simulink model "model_virtualagent_bros"  (R2016b)
settings: Solver=FixedStepDiscrete  StartTime=0.0  StopTime=inf  FixedStep=sampleTime  RelTol=1e-3
PostLoadFcn:
  | % load model parameters
  | % pname = fileparts(get_param('model_virtualagent_bros','filename'));
  | % run([pname  '\parameters_base_model_bros.m']);
  | parameters_base_model_bros;
  | 
  | % set requested state
  | set_param('model_virtualagent_bros/Requested state','Value',num2str(0));
InitFcn:
  | % load model parameters
  | % pname = fileparts(get_param('model_base_bros','filename'));
  | % run([pname  '\parameters_base_model_bros.m']);
  | parameters_base_model_bros;
  | 
  | % set requested state
  | set_param('model_virtualagent_bros/Requested state','Value',num2str(0));
StartFcn:
  | % load model parameters
  | % pname = fileparts(get_param('model_base_bros','filename'));
  | % run([pname  '\parameters_base_model_bros.m']);
  | parameters_base_model_bros;
  | 
  | % set requested state
  | set_param('model_virtualagent_bros/Requested state','Value',num2str(0));
values from neighbouring files (symbols this model uses):
  Ae_vp = [1 2;3 4]    [parameters_base_model_bros.m]
  Aim_vp = Ae_vp    [parameters_base_model_bros.m]    (also in parameters_virtualpartner_bros.m = dynamics_vp(sampleTime,m_vp,tu,td,tp,gamma*D))
  Ax = [0.0286583637244 0.0270981680387 0.0234505258969 0.0179991434705]    [data_target_signal.mat]    (also in data_target_signal3.mat = [0.0333782282668 0.0245436264839 0.0161138842629 0.007570500; data_target_signal4.mat = [0.0269405878553 0.022932388404 0.0177213023263 0.0101459636; data_target_signal5.mat = [0.0280601816416 0.0238854099083 0.0184577621273 0.010567608)
  Ay = [0.0270981680387 0.0253254894496 0.0215637914741 0.0163904070646]    [data_target_signal.mat]    (also in data_target_signal3.mat = [0.0316365733513 0.022903298684 0.0150378639378 0.0071644979; data_target_signal4.mat = [0.0262391735578 0.0220449066546 0.0169202788634 0.009702651; data_target_signal5.mat = [0.0273296180511 0.0229610462966 0.0176234498254 0.010105872)
  FFMatrix = [0 -20; 20 0]*-1    [parameters_base_model_bros.m]    (also in parameters_model_virtualpartner_bros.m = -[0 -15; 15 0]; parameters_virtualpartner_bros.m = -[0 -15; 15 0])
  Lb = 0.07    [parameters_base_model_bros.m]    (also in parameters_model_virtualpartner_bros.m; parameters_virtualpartner_bros.m)
  Lf = 0.238    [parameters_base_model_bros.m]    (also in parameters_model_virtualpartner_bros.m; parameters_virtualpartner_bros.m)
  Lu = 0.153    [parameters_base_model_bros.m]    (also in parameters_model_virtualpartner_bros.m; parameters_virtualpartner_bros.m)
  nx = [3 4 6 9]    [data_target_signal.mat]    (also in data_target_signal3.mat = [6 11 17 29]; data_target_signal4.mat = [6 11 17 29]; data_target_signal5.mat = [6 11 17 29])
  ny = [4 5 7 10]    [data_target_signal.mat]    (also in data_target_signal3.mat = [7 12 18 30]; data_target_signal4.mat = [7 12 18 30]; data_target_signal5.mat = [7 12 18 30])
  P0_vp = zeros(2,2)    [parameters_base_model_bros.m]
  phx = [-7.77441521106 -8.5348832042 -4.36104325862 -3.78796037329]    [data_target_signal.mat]    (also in data_target_signal3.mat = [3.56575266464 -2.00335535647 1.65538939475 0.759048650391]; data_target_signal4.mat = [-7.8125213649 -4.12353525545 6.3256632478 -1.21163926456]; data_target_signal5.mat = [2.80153374524 -3.20046313064 -3.48286348128 -10.5236026319])
  phy = [-0.714244784373 -3.45250659197 3.9180169666 4.93073057512]    [data_target_signal.mat]    (also in data_target_signal3.mat = [9.98760310067 -6.16453798136 -6.84315611985 5.69872885715]; data_target_signal4.mat = [6.54917483844 9.11210927212 4.8993819932 2.56946947623]; data_target_signal5.mat = [-1.40862004251 -1.67034924642 8.20266618674 -4.37156725072])
  sampleTime = 0.001    [parameters_base_model_bros.m]    (also in parameters_model_virtualpartner_bros.m; parameters_virtualpartner_bros.m)
undefined symbols (not defined in the file or in its folder): B_vp, BROS1, BROS2, C_vp
libraries: simulink x26, LibraryFM x14, VariousBlocksLibrary x6, simulink_extras x1
(part 3 of 3)

== system model_virtualagent_bros/Robot1/DataFromEtherCAT/Calculate Arrange Joint and Op Space/forward kinematics1 ==
  JointPosition_rad : Inport  PortDimensions=[2 1]
  JointVelocity_rads : Inport  Port=2  PortDimensions=[2 1]
  JointAcceleration_rads2 : Inport  Port=3  PortDimensions=[2 1]
  Je : MATLAB Function  TreatAsAtomicUnit=on
  Jedot : MATLAB Function  TreatAsAtomicUnit=on
  Product : Product  Multiplication=Matrix(*)
  calculate xddot : MATLAB Function  TreatAsAtomicUnit=on
  forward kinematics : MATLAB Function  TreatAsAtomicUnit=on
  x : Outport
  xdot : Outport  Port=2
  xddot : Outport  Port=3
  J : Outport  Port=4
  Jdot : Outport  Port=5
  wires:
  JointPosition_rad/1 -> forward kinematics/1(q), Jedot/1(q), Je/1(q)
  Je/1(Je) -> calculate xddot/3(J), Product/1, J/1
  JointVelocity_rads/1 -> calculate xddot/2(qdot), Product/2, Jedot/2(qdot)
  Jedot/1(Jedot) -> calculate xddot/4(Jdot), Jdot/1
  Product/1 -> xdot/1
  forward kinematics/1(x) -> x/1
  calculate xddot/1(xddot) -> xddot/1
  JointAcceleration_rads2/1 -> calculate xddot/1(qddot)

== system model_virtualagent_bros/Robot2/Controller_PD/at home/HoldFirstSampleOnEnable ==
  note: These blocks hold the first sample of the input
      | when the block is enabled (through the action port)
  x : Inport
  Enable : EnablePort  StatesWhenEnabling=reset
  Counter Free-Running : simulink/Sources/Counter Free-Running  NumBits=32  tsamp=-1
  Memory1 : Memory
  Signal Conversion : SignalConversion  OverrideOpt=off
  Switch : Switch  Threshold=1
  x0 : Outport
  wires:
  x/1 -> Switch/3
  Counter Free-Running/1 -> Switch/2
  Memory1/1 -> Switch/1
  Switch/1 -> Signal Conversion/1, Memory1/1
  Signal Conversion/1 -> x0/1

== system model_virtualagent_bros/Robot2/DataFromEtherCAT/Calculate Arrange Joint and Op Space/forward kinematics ==
  JointPosition_rad : Inport  PortDimensions=[2 1]
  JointVelocity_rads : Inport  Port=2  PortDimensions=[2 1]
  JointAcceleration_rads2 : Inport  Port=3  PortDimensions=[2 1]
  Je : MATLAB Function  TreatAsAtomicUnit=on
  Jedot : MATLAB Function  TreatAsAtomicUnit=on
  Product : Product  Multiplication=Matrix(*)
  calculate xddot : MATLAB Function  TreatAsAtomicUnit=on
  forward kinematics : MATLAB Function  TreatAsAtomicUnit=on
  x : Outport
  xdot : Outport  Port=2
  xddot : Outport  Port=3
  J : Outport  Port=4
  Jdot : Outport  Port=5
  wires:
  JointPosition_rad/1 -> forward kinematics/1(q), Jedot/1(q), Je/1(q)
  Je/1(Je) -> calculate xddot/3(J), Product/1, J/1
  JointVelocity_rads/1 -> calculate xddot/2(qdot), Product/2, Jedot/2(qdot)
  Jedot/1(Jedot) -> calculate xddot/4(Jdot), Jdot/1
  Product/1 -> xdot/1
  forward kinematics/1(x) -> x/1
  calculate xddot/1(xddot) -> xddot/1
  JointAcceleration_rads2/1 -> calculate xddot/1(qddot)

== system model_virtualagent_bros/Robot2/DataFromEtherCAT/Calculate Arrange Joint and Op Space/forward kinematics1 ==
  JointPosition_rad : Inport  PortDimensions=[2 1]
  JointVelocity_rads : Inport  Port=2  PortDimensions=[2 1]
  JointAcceleration_rads2 : Inport  Port=3  PortDimensions=[2 1]
  Je : MATLAB Function  TreatAsAtomicUnit=on
  Jedot : MATLAB Function  TreatAsAtomicUnit=on
  Product : Product  Multiplication=Matrix(*)
  calculate xddot : MATLAB Function  TreatAsAtomicUnit=on
  forward kinematics : MATLAB Function  TreatAsAtomicUnit=on
  x : Outport
  xdot : Outport  Port=2
  xddot : Outport  Port=3
  J : Outport  Port=4
  Jdot : Outport  Port=5
  wires:
  JointPosition_rad/1 -> forward kinematics/1(q), Jedot/1(q), Je/1(q)
  Je/1(Je) -> calculate xddot/3(J), Product/1, J/1
  JointVelocity_rads/1 -> calculate xddot/2(qdot), Product/2, Jedot/2(qdot)
  Jedot/1(Jedot) -> calculate xddot/4(Jdot), Jdot/1
  Product/1 -> xdot/1
  forward kinematics/1(x) -> x/1
  calculate xddot/1(xddot) -> xddot/1
  JointAcceleration_rads2/1 -> calculate xddot/1(qddot)

== matlab function model_virtualagent_bros/Robot2/Controller_PD/PD + nonlin (op space)/Jt ==
  data: x input; J input; y output
function y = Jt(x,J)

y = J.'*x;

== matlab function model_virtualagent_bros/Experiment & Haptics/CalculateTrialPerformanceMSE/Calc_RMSE_BROS1 ==
  data: error input; RMSE output
function RMSE = RMSE(error)
% calculate the mean-squared error

persistent N; % number of samples, counter
persistent SSE; % sum of squared of error
if isempty(N), N = 0; end
if isempty(SSE), SSE = 0; end

N = N+1; % new datapoint, increase sample counter

SSE = SSE + norm(error)^2;
RMSE = sqrt(SSE / N);

== matlab function model_virtualagent_bros/Robot1/DataFromEtherCAT/Calculate Arrange Joint and Op Space/Condition number ==
  data: J input; C output
function C = conditioning(J)
%#codegen

C = norm(J)*norm(pinv(J));

== matlab function model_virtualagent_bros/Robot1/DataFromEtherCAT/Calculate Arrange Joint and Op Space/forward kinematics1/Je ==
  data: q input; Je output size=[2 2]; Lf parameter; Lu parameter; Lb parameter
function Je = Je( q, Lf, Lu, Lb)
%#codegen

% Calculate the Jacobian for this particular device configuration.
% Note that the function func_eq_Je needs to be in the libraries/kinematis_functions folder

% jacobians
Je = func_eq_Je(q(1),q(2),Lf,Lu,Lb);

== matlab function model_virtualagent_bros/Robot1/DataFromEtherCAT/Calculate Arrange Joint and Op Space/forward kinematics1/Jedot ==
  data: q input; qdot input; Jedot output size=[2 2]; Lf parameter; Lu parameter; Lb parameter
function Jedot = Jedot( q, qdot, Lf, Lu, Lb)
%#codegen

% Calculate the time derivative of the Jacobian for this particular device configuration.
% Note that the function func_eq_Je needs to be in the libraries/kinematis_functions folder


% jacobians
Jedot = func_eq_Jedot(q(1),q(2),qdot(1),qdot(2),Lf,Lu,Lb);

== matlab function model_virtualagent_bros/Robot1/DataFromEtherCAT/Calculate Arrange Joint and Op Space/forward kinematics1/calculate xddot ==
  data: qddot input; qdot input size=[2 1]; J input; xddot output size=[2 1]; Jdot input
function xddot = calc_xddot(qddot, qdot, J, Jdot)
%#codegen

xddot = J*qddot + Jdot*qdot;

== matlab function model_virtualagent_bros/Robot2/Controller_PD/PD + nonlin (op space)/nonlinear compensation ==
  data: J input; Jdot input; qdot input; tau output; RobotStruct parameter
function tau = n(J,Jdot,qdot,RobotStruct)
% mass matrix
phat = RobotStruct.DynModParams;

% select parameters
me = phat(3);
Fs1 = phat(4);
Fv1 = phat(5);
Fs2 = phat(6);
Fv2 = phat(7);

% % jacobians
% J = func_eq_Je(q(1),q(2),Lf,Lu,Lb);
% Jdot = func_eq_Jedot(q(1),q(2),qdot(1),qdot(2),Lf,Lu,Lb);

% calculate joint space mass matrix;
p = [me;Fs1;Fv1;Fs2;Fv2];

% psi 
Psi = [(J'*Jdot)*qdot [ssign(qdot(1)) qdot(1); 0 0] [0 0; ssign(qdot(2)) qdot(2)]];

% torque
tau = Psi*p;

function x = ssign(u,b)
%% x = ssign(u,b)
% soft sign
if nargin < 2
    b = 4;
end

x = 2./(1+exp(-b*u))-1;

== matlab function model_virtualagent_bros/Experiment & Haptics/Target position ==
  data: time input; T input; time_rand input; p output; nx parameter; ny parameter; Ax parameter; Ay parameter; phx parameter; phy parameter
function p  = msin_target (time, T, time_rand, nx, ny, Ax, Ay, phx, phy) 

% prepare frequencies
dw = 2*pi/T; %w0 depends on trial duration
wx = dw*nx;
wy = dw*ny;

% calculate x and y
px = 0;
py = 0;

% randomization
% for every multiple of 20, mirror x, y, or xy
% nRand = 0: no mirror
% nRand = 1: x mirror
% nRand = 2: y mirror
% nRand = 3: xy mirror
nRand = floor(time_rand/20);
if nRand > 3, nRand = 3; end

% add random starting time (semi-randomization)
time = time + mod(time_rand,20.0);

% calculate sum-of-sines
for i = 1:length(wx)
    px = px + Ax(i)*sin(wx(i)*time+phx(i));
    py = py + Ay(i)*sin(wy(i)*time+phy(i));
end

p = [px; py];

% mirror position, based on nRand
switch nRand
    case 0
        % do nothing
    case 1
        p = [-1;1].*p;
    case 2
        p = [1;-1].*p;
    case 3
        p = [-1;-1].*p;
    otherwise
        % do nothing
end
end

== matlab function model_virtualagent_bros/Robot1/DataFromEtherCAT/Calculate Arrange Joint and Op Space/forward kinematics/forward kinematics ==
  data: q input; x output size=[2 1]; Lf parameter; Lu parameter; Lb parameter
function x = FK(q, Lf, Lu, Lb)
%#codegen

% Calculate the endpoint position (forward kinematics)
% Note that the function func_eq_FK needs to be in the libraries/kinematis_functions folder


x = func_eq_FK(q(1),q(2),Lf,Lu,Lb);

== matlab function model_virtualagent_bros/Robot1/DataFromEtherCAT/Calculate Arrange Joint and Op Space/forward kinematics1/forward kinematics ==
  data: q input; x output size=[2 1]; Lf parameter; Lu parameter; Lb parameter
function x = FK(q, Lf, Lu, Lb)
%#codegen

% Calculate the endpoint position (forward kinematics)
% Note that the function func_eq_FK needs to be in the libraries/kinematis_functions folder


x = func_eq_FK(q(1),q(2),Lf,Lu,Lb);

== matlab function model_virtualagent_bros/Robot1/DataToEtherCAT/FTSensorError/MATLAB Function ==
  data: ForcesTorques input; e output; MaxForcesTorques input
function e = fcn(ForcesTorques, MaxForcesTorques)

% throw error when any of the forces/torques go over a max allowable value
if any(abs(ForcesTorques) > MaxForcesTorques) 
    e = 1;
else
    e = 0;
end

== matlab function model_virtualagent_bros/Robot1/Controller_PD/PD + nonlin (op space)/invJ1 ==
  data: x input; J input; y output
function y = invJ(x,J)

y = J.'*x;

== matlab function model_virtualagent_bros/Robot2/DataFromEtherCAT/Calculate Arrange Joint and Op Space/Condition number ==
  data: J input; C output
function C = conditioning(J)
%#codegen

C = norm(J)*norm(pinv(J));

== matlab function model_virtualagent_bros/Robot2/DataFromEtherCAT/Calculate Arrange Joint and Op Space/IK all joints ==
  data: x input; q_all output; Lf parameter; Lu parameter; Lb parameter
function q_all = IK_all(x,Lf,Lu,Lb)
%#codegen

q_all = func_eqs_IK_all(x(1),x(2),Lf,Lu,Lb);

if any(isnan(q_all)) || any(isinf(q_all))
    q_all = zeros(5,1);
end

== matlab function model_virtualagent_bros/Robot2/DataFromEtherCAT/Calculate Arrange Joint and Op Space/forward kinematics/Je ==
  data: q input; Je output size=[2 2]; Lf parameter; Lu parameter; Lb parameter
function Je = Je( q, Lf, Lu, Lb)
%#codegen

% Calculate the Jacobian for this particular device configuration.
% Note that the function func_eq_Je needs to be in the libraries/kinematis_functions folder

% jacobians
Je = func_eq_Je(q(1),q(2),Lf,Lu,Lb);

== matlab function model_virtualagent_bros/Robot2/DataFromEtherCAT/Calculate Arrange Joint and Op Space/forward kinematics/Jedot ==
  data: q input; qdot input; Jedot output size=[2 2]; Lf parameter; Lu parameter; Lb parameter
function Jedot = Jedot( q, qdot, Lf, Lu, Lb)
%#codegen

% Calculate the time derivative of the Jacobian for this particular device configuration.
% Note that the function func_eq_Je needs to be in the libraries/kinematis_functions folder


% jacobians
Jedot = func_eq_Jedot(q(1),q(2),qdot(1),qdot(2),Lf,Lu,Lb);

== matlab function model_virtualagent_bros/Robot1/DataFromEtherCAT/Calculate Arrange Joint and Op Space/forward kinematics/Je ==
  data: q input; Je output size=[2 2]; Lf parameter; Lu parameter; Lb parameter
function Je = Je( q, Lf, Lu, Lb)
%#codegen

% Calculate the Jacobian for this particular device configuration.
% Note that the function func_eq_Je needs to be in the libraries/kinematis_functions folder

% jacobians
Je = func_eq_Je(q(1),q(2),Lf,Lu,Lb);

== matlab function model_virtualagent_bros/Robot1/DataFromEtherCAT/Calculate Arrange Joint and Op Space/forward kinematics/Jedot ==
  data: q input; qdot input; Jedot output size=[2 2]; Lf parameter; Lu parameter; Lb parameter
function Jedot = Jedot( q, qdot, Lf, Lu, Lb)
%#codegen

% Calculate the time derivative of the Jacobian for this particular device configuration.
% Note that the function func_eq_Je needs to be in the libraries/kinematis_functions folder


% jacobians
Jedot = func_eq_Jedot(q(1),q(2),qdot(1),qdot(2),Lf,Lu,Lb);

== matlab function model_virtualagent_bros/Robot1/DataFromEtherCAT/FTSensor_K6D27/CorrectOffset ==
  data: u_in input; u_out output; reset input; corrected output
function [u_out,corrected] = CorrectOffset(u_in,reset)
%#codegen

persistent data_ offset_ counter_ corrected_;
N = 1000;

% initialize
if isempty(data_)
    data_ = zeros(size(u_in,1), N);
    offset_ = zeros(size(u_in));
    counter_ = 1;
    corrected_ = 0;
end

if (counter_ <= N)
    data_(:,counter_) = u_in;
end

counter_ = counter_ + 1;
if reset
    counter_ = 1;
end

% calculate mean
if counter_ == N
    corrected_ = 1;
    offset_ = mean(data_,2);
end

corrected = corrected_;
u_out = u_in - offset_;

== matlab function model_virtualagent_bros/Robot2/DataFromEtherCAT/Calculate Arrange Joint and Op Space/forward kinematics/calculate xddot ==
  data: qddot input; qdot input size=[2 1]; J input; xddot output size=[2 1]; Jdot input
function xddot = calc_xddot(qddot, qdot, J, Jdot)
%#codegen

xddot = J*qddot + Jdot*qdot;

== matlab function model_virtualagent_bros/Robot1/DataFromEtherCAT/Calculate Arrange Joint and Op Space/IK all joints ==
  data: x input; q_all output; Lf parameter; Lu parameter; Lb parameter
function q_all = IK_all(x,Lf,Lu,Lb)
%#codegen

q_all = func_eqs_IK_all(x(1),x(2),Lf,Lu,Lb);

if any(isnan(q_all)) || any(isinf(q_all))
    q_all = zeros(5,1);
end

== matlab function model_virtualagent_bros/Robot1/DataFromEtherCAT/Calculate Arrange Joint and Op Space/forward kinematics/calculate xddot ==
  data: qddot input; qdot input size=[2 1]; J input; xddot output size=[2 1]; Jdot input
function xddot = calc_xddot(qddot, qdot, J, Jdot)
%#codegen

xddot = J*qddot + Jdot*qdot;

== matlab function model_virtualagent_bros/Robot2/DataFromEtherCAT/Calculate Arrange Joint and Op Space/forward kinematics/forward kinematics ==
  data: q input; x output size=[2 1]; Lf parameter; Lu parameter; Lb parameter
function x = FK(q, Lf, Lu, Lb)
%#codegen

% Calculate the endpoint position (forward kinematics)
% Note that the function func_eq_FK needs to be in the libraries/kinematis_functions folder


x = func_eq_FK(q(1),q(2),Lf,Lu,Lb);

== matlab function model_virtualagent_bros/Robot1/Controller_PD/PD + nonlin (op space)/nonlinear compensation ==
  data: J input; Jdot input; qdot input; tau output; RobotStruct parameter
function tau = n(J,Jdot,qdot,RobotStruct)
% mass matrix
phat = RobotStruct.DynModParams;

% select parameters
me = phat(3);
Fs1 = phat(4);
Fv1 = phat(5);
Fs2 = phat(6);
Fv2 = phat(7);

% % jacobians
% J = func_eq_Je(q(1),q(2),Lf,Lu,Lb);
% Jdot = func_eq_Jedot(q(1),q(2),qdot(1),qdot(2),Lf,Lu,Lb);

% calculate joint space mass matrix;
p = [me;Fs1;Fv1;Fs2;Fv2];

% psi 
Psi = [(J'*Jdot)*qdot [ssign(qdot(1)) qdot(1); 0 0] [0 0; ssign(qdot(2)) qdot(2)]];

% torque
tau = Psi*p;

function x = ssign(u,b)
%% x = ssign(u,b)
% soft sign
if nargin < 2
    b = 8;
end

x = 2./(1+exp(-b*u))-1;

== matlab function model_virtualagent_bros/Robot2/DataFromEtherCAT/Calculate Arrange Joint and Op Space/forward kinematics1/Je ==
  data: q input; Je output size=[2 2]; Lf parameter; Lu parameter; Lb parameter
function Je = Je( q, Lf, Lu, Lb)
%#codegen

% Calculate the Jacobian for this particular device configuration.
% Note that the function func_eq_Je needs to be in the libraries/kinematis_functions folder

% jacobians
Je = func_eq_Je(q(1),q(2),Lf,Lu,Lb);

== matlab function model_virtualagent_bros/Robot2/DataFromEtherCAT/Calculate Arrange Joint and Op Space/forward kinematics1/Jedot ==
  data: q input; qdot input; Jedot output size=[2 2]; Lf parameter; Lu parameter; Lb parameter
function Jedot = Jedot( q, qdot, Lf, Lu, Lb)
%#codegen

% Calculate the time derivative of the Jacobian for this particular device configuration.
% Note that the function func_eq_Je needs to be in the libraries/kinematis_functions folder


% jacobians
Jedot = func_eq_Jedot(q(1),q(2),qdot(1),qdot(2),Lf,Lu,Lb);

== matlab function model_virtualagent_bros/Robot2/DataFromEtherCAT/Calculate Arrange Joint and Op Space/forward kinematics1/calculate xddot ==
  data: qddot input; qdot input size=[2 1]; J input; xddot output size=[2 1]; Jdot input
function xddot = calc_xddot(qddot, qdot, J, Jdot)
%#codegen

xddot = J*qddot + Jdot*qdot;

== matlab function model_virtualagent_bros/Robot2/DataFromEtherCAT/Calculate Arrange Joint and Op Space/forward kinematics1/forward kinematics ==
  data: q input; x output size=[2 1]; Lf parameter; Lu parameter; Lb parameter
function x = FK(q, Lf, Lu, Lb)
%#codegen

% Calculate the endpoint position (forward kinematics)
% Note that the function func_eq_FK needs to be in the libraries/kinematis_functions folder


x = func_eq_FK(q(1),q(2),Lf,Lu,Lb);

== matlab function model_virtualagent_bros/Robot2/DataFromEtherCAT/FTSensor_K6D27/CorrectOffset ==
  data: u_in input; u_out output; reset input; corrected output
function [u_out,corrected] = CorrectOffset(u_in,reset)
%#codegen

persistent data_ offset_ counter_ corrected_;
N = 1000;

% initialize
if isempty(data_)
    data_ = zeros(size(u_in,1), N);
    offset_ = zeros(size(u_in));
    counter_ = 1;
    corrected_ = 0;
end

if (counter_ <= N)
    data_(:,counter_) = u_in;
end

counter_ = counter_ + 1;
if reset
    counter_ = 1;
end

% calculate mean
if counter_ == N
    corrected_ = 1;
    offset_ = mean(data_,2);
end

corrected = corrected_;
u_out = u_in - offset_;

== matlab function model_virtualagent_bros/Robot2/DataFromEtherCAT/FTSensor_K6D27/SensorToOperationalSpace ==
  data: q_all input; Fs input; FTOpSpace output; transmatside input
function FTOpSpace = ForceSensorToOperationalSpace(q_all,Fs,transmatside)
%#codegen
q1 = q_all(1);
q2 = q_all(2);
q4 = q_all(4);
q5 = q_all(5);

% based on which arm the force sensor is connected
switch transmatside
    case 1
        alpha = pi-q2;   
        beta = q1+alpha-pi/2;
        R0 = rotmat(beta);
        R = blkdiag(R0,R0); % transform forces and moments
    case 2
        alpha = -(pi - q4);
        beta = q5+alpha-pi/2;
        R0 = rotmat(beta);
        R = blkdiag(R0,R0); % transform forces and moments
    otherwise
        R = eye(length(Fs));
end

% transform force
FTOpSpace = R*Fs;

function R = rotmat(q)

R = [cos(q) -sin(q) 0;...
      sin(q)  cos(q) 0;...
      0       0      1];

== matlab function model_virtualagent_bros/Robot2/DataToEtherCAT/CreateSingleErrorValue1/ErrorToPower2 ==
  data: u input; e output
function e = errorToPowerOf2(u)

e = (2.^(0:length(u)-1))*u;

== matlab function model_virtualagent_bros/Robot2/DataToEtherCAT/CreateSingleErrorValue2/ErrorToPower2 ==
  data: u input; e output
function e = errorToPowerOf2(u)

e = (2.^(0:length(u)-1))*u;

== matlab function model_virtualagent_bros/Robot2/DataToEtherCAT/FTSensorError/MATLAB Function ==
  data: ForcesTorques input; e output; MaxForcesTorques input
function e = fcn(ForcesTorques, MaxForcesTorques)

% throw error when any of the forces/torques go over a max allowable value
if any(abs(ForcesTorques) > MaxForcesTorques) 
    e = 1;
else
    e = 0;
end

== matlab function model_virtualagent_bros/Robot2/DataToEtherCAT/WorkspacePositionGuard/CheckInternalAngles ==
  data: theta input; angleError output
function angleError = checkInternalErrors(theta)
%#codegen


angleError = 0;
if any(theta([2 4]) >= 0.95*pi)
    angleError = 1;
end

== matlab function model_virtualagent_bros/Robot2/DataToEtherCAT/WorkspacePositionGuard/EndpointPositionGuard ==
  data: correctState input; xe input; error output
function error = fcn(correctState, xe)
%#codegen


error = 0;

% only check workspace boundaries after homing state is done
if ~correctState 
    return; 
end

% x0 = 0;
% y0 = 0.2354;
% a = 0.11;
% b = 0.08;

% workspace (see design document)
x0 = 0;
y0 = 0.25024;
a = 0.1746;
b = 0.13;%0.1048;

% check if endpoint is outside a predefined ellipse
x = xe(1);
y = xe(2);

% workspace is defined as an ellipse
e = (x-x0)^2 / a^2 + (y-y0)^2 / b^2;

% if is larger than 1, the endpoint is outside the workspace
if e > 1
    error = 1;
end

== matlab function model_virtualagent_bros/Experiment & Haptics/CalculateTrialPerformanceMSE/Calc_RMSE_BROS2 ==
  data: error input; RMSE output
function RMSE = RMSE(error)
% calculate the mean-squared error

persistent N; % number of samples, counter
persistent SSE; % sum of squared of error
if isempty(N), N = 0; end
if isempty(SSE), SSE = 0; end

N = N+1; % new datapoint, increase sample counter

SSE = SSE + norm(error)^2;
RMSE = sqrt(SSE / N);

== matlab function model_virtualagent_bros/Robot1/DataToEtherCAT/CreateSingleErrorValue2/ErrorToPower2 ==
  data: u input; e output
function e = errorToPowerOf2(u)

e = (2.^(0:length(u)-1))*u;

== matlab function model_virtualagent_bros/Robot1/DataToEtherCAT/CreateSingleErrorValue1/ErrorToPower2 ==
  data: u input; e output
function e = errorToPowerOf2(u)

e = (2.^(0:length(u)-1))*u;

== matlab function model_virtualagent_bros/Robot1/DataFromEtherCAT/FTSensor_K6D27/SensorToOperationalSpace ==
  data: q_all input; Fs input; FTOpSpace output; transmatside input
function FTOpSpace = ForceSensorToOperationalSpace(q_all,Fs,transmatside)
%#codegen
q1 = q_all(1);
q2 = q_all(2);
q4 = q_all(4);
q5 = q_all(5);

% based on which arm the force sensor is connected
switch transmatside
    case 1
        alpha = pi-q2;   
        beta = q1+alpha-pi/2;
        R0 = rotmat(beta);
        R = blkdiag(R0,R0); % transform forces and moments
    case 2
        alpha = -(pi - q4);
        beta = q5+alpha-pi/2;
        R0 = rotmat(beta);
        R = blkdiag(R0,R0); % transform forces and moments
    otherwise
        R = eye(length(Fs));
end

% transform force
FTOpSpace = R*Fs;

function R = rotmat(q)

R = [cos(q) -sin(q) 0;...
      sin(q)  cos(q) 0;...
      0       0      1];

== matlab function model_virtualagent_bros/Experiment & Haptics/Admittance // Virtual model1/Virtual Model/Virtual model ==
  data: divTs input; x1 output; xdot1 output; xddot1 output; x2 output size=[2 1]; xdot2 output; xddot2 output; M_v input; B_v input; F1 input; F2 input; x0_1 input; x0_2 input; x1_nompos input; x2_nompos input; Kp_s input; Kd_s input; isConnected input; FFMatrix input; doForceField input; Ae_vp input; Aim_vp input; B_vp input; C_vp input; L_vp input; P0_vp input; enableVirtualAgents input; Fconn_prev1 input; Fconn_prev2 input; x1_prev input size=2; xdot1_prev input size=2; x2_prev input; xdot2_prev input; sampleTime parameter; Fs1 output; Fs2 output
function [x1,xdot1,xddot1,x2,xdot2,xddot2, Fs1, Fs2] = AC(divTs, M_v, B_v, F1, F2, x0_1, x0_2, x1_nompos, x2_nompos,...
                                                Kp_s, Kd_s, isConnected,...
                                                FFMatrix,doForceField,...
                                                Ae_vp,Aim_vp,B_vp,C_vp,L_vp,P0_vp,enableVirtualAgents,...
                                                Fconn_prev1,Fconn_prev2,x1_prev,xdot1_prev,x2_prev,xdot2_prev,sampleTime)                                          
%% function [x1,xdot1,xddot1,x2,xdot2,xddot2] = AC(divTs, M_v, B_v, F1, F2, x0_1, x0_2, x1_nompos, x2_nompos,...
%                                                 Kp_s, Kd_s, isConnected,...
%                                                 FFMatrix,doForceField,...
%                                                 Ae_vp,Aim_vp,B_vp,C_vp,L_vp,P0_vp,enableVirtualAgents,...
%                                                 x1_prev,xdot1_prev,x2_prev,xdot2_prev,sampleTime)                                            



% constants & limits
div_Ts = max(1,divTs);
Ts = sampleTime/div_Ts;
maxRadius = 0.1;
maxVel = 2.0;
maxAcc = 100.0;
maxForceConnection = 50;
b_b = 0.5; % damping on boundary

% persistents
persistent x1_prev_tmp;
persistent x2_prev_tmp;
persistent onBoundary1;
persistent onBoundary2;
% persistent x_vp1;
% persistent x_vp2;

if isempty(x1_prev_tmp), x1_prev_tmp = x0_1;
else, x1_prev_tmp = x1_prev; end 

if isempty(x2_prev_tmp), x2_prev_tmp = x0_2;
else, x2_prev_tmp = x2_prev; end 

if isempty(onBoundary1), onBoundary1 = 0; end
if isempty(onBoundary2), onBoundary2 = 0; end

% lower bounds to mass and damping
m_v = max(0.2,M_v); %lower bound M_v
b_v = max(0,B_v);

if length(m_v) == 1
    m_v1 = m_v;
    m_v2 = m_v;
else
    m_v1 = m_v(1);
    m_v2 = m_v(2);
end

if length(b_v) == 1
    b_v1 = b_v;
    b_v2 = b_v;
else
    b_v1 = b_v(1);
    b_v2 = b_v(2);
end

% assign previous  values to x1, x2, xdot1 etc
x1 = x1_prev;
x2 = x2_prev;
xdot1 = xdot1_prev;
xdot2 = xdot1_prev;
xddot1 = [0;0];
xddot2 = [0;0];

% virtual agent dynamics
x_vp1 = [0;0];
xdot_vp1 = [0;0];
x_vp2 = [0;0];
xdot_vp2 = [0;0];




% perform integration of virtual dynamics
% using semi-implicit Euler integration
for ii = 1:div_Ts
    
    % spring force
    Fs1 = [0;0];
    Fs2 = [0;0];
    
    % calculate connection force for connection to virtual agent 
    if (enableVirtualAgents(1) == 1)
        % spring force virtual agent 1
        Fs1 = Kp_s*(x_vp1 - x1_prev) + Kd_s*(xdot_vp1 - xdot1_prev);
    end
    
    if (enableVirtualAgents(2) == 1)
        % spring force virtual agent 2
        Fs2 = Kp_s*(x_vp2 - x2_prev) + Kd_s*(xdot_vp2 - xdot2_prev);
    end
    
    % if no virtual agents used, just calculate spring force for human-human connection
    if all(enableVirtualAgents == 0)
        Fs1 = Kp_s*(x2_prev - x1_prev) + Kd_s*(xdot2_prev - xdot1_prev);
        Fs2 = -Fs1;
    end

    % limit connection force
    Fs1 = limit(Fs1,maxForceConnection);
    Fs2 = limit(Fs2,maxForceConnection);
    
    % calculate admittance model dynamics acceleration
    
    % BROS 1
    xddot1 = (F1 + isConnected*Fs1 + doForceField*FFMatrix*xdot1_prev - b_v1*xdot1_prev - onBoundary1*b_b*xdot1_prev)/m_v1;
    xddot1 = limit(xddot1,maxAcc);

    % BROS 2
    xddot2 = (F2 + isConnected*Fs2 + doForceField*FFMatrix*xdot2_prev - b_v2*xdot2_prev - onBoundary2*b_b*xdot2_prev)/m_v2;
    xddot2 = limit(xddot2,maxAcc);

    % acc -> vel
    % BROS 1
    xdot1 = xdot1_prev + xddot1*Ts;
    [xdot1,lim_vel] = limit(xdot1,maxVel);

    if (lim_vel)
        xddot1 = [0;0];
    end

    % BROS 2
    xdot2 = xdot2_prev + xddot2*Ts;
    [xdot2,lim_vel] = limit(xdot2,maxVel);

    if (lim_vel)
        xddot2 = [0;0];
    end

    % vel -> pos
    % BROS 1
    x1 = x1_prev_tmp + xdot1*Ts;

    [x1,lim_pos] = limit(x1-x1_nompos,maxRadius);
    if (lim_pos)
        onBoundary1 = 1;
        unitVec = x1/norm(x1);
        xdot1 = xdot1 - dot(unitVec,xdot1)*unitVec;     % remove normal component
        xddot1 = xddot1 - dot(unitVec,xddot1)*unitVec;  % remove normal component 
    else
        onBoundary1 = 0;
    end
    x1 = x1 + x1_nompos;

    % BROS 2
    x2 = x2_prev_tmp + xdot2*Ts;

    [x2,lim_pos] = limit(x2-x2_nompos,maxRadius);
    if (lim_pos)
        onBoundary2 = 1;
        unitVec = x2/norm(x2);
        xdot2 = xdot2 - dot(unitVec,xdot2)*unitVec;     % remove normal component
        xddot2 = xddot2 - dot(unitVec,xddot2)*unitVec;  % remove normal component 
    else
        onBoundary2 = 0;
    end
    x2 = x2 + x2_nompos;
    
    x1_prev_tmp = x1;
    x2_prev_tmp = x2;
    xdot1_prev = xdot1;
    xdot2_prev = xdot2;
end

end

% limit
function [y,lim] = limit(x,maxVal)
    vecLen = norm(x);
    if vecLen > maxVal
        y = x / vecLen * maxVal;
        lim = 1; 
    else
        y = x;
        lim = 0;
    end
end

== matlab function model_virtualagent_bros/Robot1/DataToEtherCAT/WorkspacePositionGuard/CheckInternalAngles ==
  data: theta input; angleError output
function angleError = checkInternalErrors(theta)
%#codegen


angleError = 0;
if any(theta([2 4]) >= 0.95*pi)
    angleError = 1;
end

== matlab function model_virtualagent_bros/Robot1/DataToEtherCAT/WorkspacePositionGuard/EndpointPositionGuard ==
  data: correctState input; xe input; error output
function error = fcn(correctState, xe)
%#codegen


error = 0;

% only check workspace boundaries after homing state is done
if ~correctState 
    return; 
end

% x0 = 0;
% y0 = 0.2354;
% a = 0.11;
% b = 0.08;

% workspace (see design document)
x0 = 0;
y0 = 0.25024;
a = 0.1746;
b = 0.13;%0.1048;

% check if endpoint is outside a predefined ellipse
x = xe(1);
y = xe(2);

% workspace is defined as an ellipse
e = (x-x0)^2 / a^2 + (y-y0)^2 / b^2;

% if is larger than 1, the endpoint is outside the workspace
if e > 1
    error = 1;
end
